simulink model "EHB_speedgoat_R2020a_V1"  (R2020a)
settings: Solver=FixedStepDiscrete  StartTime=0.0  StopTime=inf  FixedStep=0.001  RelTol=1e-3  EnableMultiTasking=on
model workspace (MAT data in the model file):
  A : Simulink.Signal (value not decoded)
  B : Simulink.Signal (value not decoded)
  C : Simulink.Signal (value not decoded)
  D : Simulink.Signal (value not decoded)
  E : Simulink.Signal (value not decoded)
  calin = [-9.96 -7.98 -5.98 -3.99 -1.994 0 1.995 3.992 5.99 7.98 9.97]
  calout = [-10 -8 -6 -4 -2 0 2 4 6 8 10]
symbols that are objects in the model workspace (value not decoded): C, D
undefined symbols (not defined in the file): Com1, none, ts_IO612
libraries: simulink x1436, xpcethercatlib x1223, yisutbxlib_utilities x256, xpcutilitieslib x156, hdlsllib x145, canmsglib x46, speedgoatlib_IO602_4 x11, speedgoatlib_IO611 x7, slrttcplib x4, CanManageLib x3, slrtlib x3, xpcseriallib x2
(part 30 of 30)

== system EHB_speedgoat_R2020a_V1/保留/YS4008/YS4008_M_6/YS4008_M/FIU_CH6/Protect ==
  KL30_In : Inport
  KL31_In : Inport  Port=2
  COM_In : Inport  Port=3
  Open_In : Inport  Port=4
  Compare To Constant{,2,12,14} (4 alike) : simulink/Logic and Bit Operations/Compare To Constant  relop===  const=1  OutDataTypeStr=boolean
  Compare To Constant{1,3..11,13,15} (12 alike) : simulink/Logic and Bit Operations/Compare To Constant  relop===  const=0  OutDataTypeStr=boolean
  Logical Operator{,1..3} (4 alike) : Logic  Inputs=4  AllPortsSameDT=off  OutDataTypeStr=boolean
  KL30_Out : Outport
  KL31_Out : Outport  Port=2
  COM_Out : Outport  Port=3
  Open_Out : Outport  Port=4
  wires:
  [Open_In] -> Compare To Constant14/1
  [COM_In] -> Compare To Constant13/1
  [KL31_In] -> Compare To Constant10/1
  [KL30_In] -> Compare To Constant8/1
  [Open_In] -> Compare To Constant15/1
  [COM_In] -> Compare To Constant12/1
  [KL31_In] -> Compare To Constant11/1
  [KL30_In] -> Compare To Constant7/1
  [COM_In] -> Compare To Constant5/1
  [KL31_In] -> Compare To Constant2/1
  [KL30_In] -> Compare To Constant1/1
  [Open_In] -> Compare To Constant6/1
  [COM_In] -> Compare To Constant4/1
  [KL31_In] -> Compare To Constant3/1
  [KL30_In] -> Compare To Constant/1
  [Open_In] -> Compare To Constant9/1
  Logical Operator/1 -> [KL30_Out]
  Logical Operator3/1 -> [Open_Out]
  Logical Operator2/1 -> [COM_Out]
  Logical Operator1/1 -> [KL31_Out]
  [Open_Out] -> Open_Out/1
  Compare To Constant7/1 -> Logical Operator2/1
  Compare To Constant11/1 -> Logical Operator2/2
  Compare To Constant12/1 -> Logical Operator2/3
  Compare To Constant15/1 -> Logical Operator2/4
  Compare To Constant14/1 -> Logical Operator3/4
  Compare To Constant13/1 -> Logical Operator3/3
  Compare To Constant10/1 -> Logical Operator3/2
  Compare To Constant8/1 -> Logical Operator3/1
  Compare To Constant1/1 -> Logical Operator1/1
  Compare To Constant2/1 -> Logical Operator1/2
  Compare To Constant5/1 -> Logical Operator1/3
  Compare To Constant6/1 -> Logical Operator1/4
  Compare To Constant9/1 -> Logical Operator/4
  Open_In/1 -> [Open_In]
  [KL31_Out] -> KL31_Out/1
  [KL30_Out] -> KL30_Out/1
  [COM_Out] -> COM_Out/1
  Compare To Constant4/1 -> Logical Operator/3
  Compare To Constant3/1 -> Logical Operator/2
  KL31_In/1 -> [KL31_In]
  KL30_In/1 -> [KL30_In]
  COM_In/1 -> [COM_In]
  Compare To Constant/1 -> Logical Operator/1

== system EHB_speedgoat_R2020a_V1/保留/YS4008/YS4008_M_6/YS4008_M/FIU_CH7/Protect ==
  KL30_In : Inport
  KL31_In : Inport  Port=2
  COM_In : Inport  Port=3
  Open_In : Inport  Port=4
  Compare To Constant{,2,12,14} (4 alike) : simulink/Logic and Bit Operations/Compare To Constant  relop===  const=1  OutDataTypeStr=boolean
  Compare To Constant{1,3..11,13,15} (12 alike) : simulink/Logic and Bit Operations/Compare To Constant  relop===  const=0  OutDataTypeStr=boolean
  Logical Operator{,1..3} (4 alike) : Logic  Inputs=4  AllPortsSameDT=off  OutDataTypeStr=boolean
  KL30_Out : Outport
  KL31_Out : Outport  Port=2
  COM_Out : Outport  Port=3
  Open_Out : Outport  Port=4
  wires:
  Compare To Constant/1 -> Logical Operator/1
  COM_In/1 -> [COM_In]
  KL30_In/1 -> [KL30_In]
  KL31_In/1 -> [KL31_In]
  Compare To Constant3/1 -> Logical Operator/2
  Compare To Constant4/1 -> Logical Operator/3
  [COM_Out] -> COM_Out/1
  [KL30_Out] -> KL30_Out/1
  [KL31_Out] -> KL31_Out/1
  Open_In/1 -> [Open_In]
  Compare To Constant9/1 -> Logical Operator/4
  Compare To Constant6/1 -> Logical Operator1/4
  Compare To Constant5/1 -> Logical Operator1/3
  Compare To Constant2/1 -> Logical Operator1/2
  Compare To Constant1/1 -> Logical Operator1/1
  Compare To Constant8/1 -> Logical Operator3/1
  Compare To Constant10/1 -> Logical Operator3/2
  Compare To Constant13/1 -> Logical Operator3/3
  Compare To Constant14/1 -> Logical Operator3/4
  Compare To Constant15/1 -> Logical Operator2/4
  Compare To Constant12/1 -> Logical Operator2/3
  Compare To Constant11/1 -> Logical Operator2/2
  Compare To Constant7/1 -> Logical Operator2/1
  [Open_Out] -> Open_Out/1
  Logical Operator1/1 -> [KL31_Out]
  Logical Operator2/1 -> [COM_Out]
  Logical Operator3/1 -> [Open_Out]
  Logical Operator/1 -> [KL30_Out]
  [Open_In] -> Compare To Constant9/1
  [KL30_In] -> Compare To Constant/1
  [KL31_In] -> Compare To Constant3/1
  [COM_In] -> Compare To Constant4/1
  [Open_In] -> Compare To Constant6/1
  [KL30_In] -> Compare To Constant1/1
  [KL31_In] -> Compare To Constant2/1
  [COM_In] -> Compare To Constant5/1
  [KL30_In] -> Compare To Constant7/1
  [KL31_In] -> Compare To Constant11/1
  [COM_In] -> Compare To Constant12/1
  [Open_In] -> Compare To Constant15/1
  [KL30_In] -> Compare To Constant8/1
  [KL31_In] -> Compare To Constant10/1
  [COM_In] -> Compare To Constant13/1
  [Open_In] -> Compare To Constant14/1

== system EHB_speedgoat_R2020a_V1/保留/YS4008/YS4008_M_6/YS4008_M/FIU_CH8/Protect ==
  KL30_In : Inport
  KL31_In : Inport  Port=2
  COM_In : Inport  Port=3
  Open_In : Inport  Port=4
  Compare To Constant{,2,12,14} (4 alike) : simulink/Logic and Bit Operations/Compare To Constant  relop===  const=1  OutDataTypeStr=boolean
  Compare To Constant{1,3..11,13,15} (12 alike) : simulink/Logic and Bit Operations/Compare To Constant  relop===  const=0  OutDataTypeStr=boolean
  Logical Operator{,1..3} (4 alike) : Logic  Inputs=4  AllPortsSameDT=off  OutDataTypeStr=boolean
  KL30_Out : Outport
  KL31_Out : Outport  Port=2
  COM_Out : Outport  Port=3
  Open_Out : Outport  Port=4
  wires:
  [Open_In] -> Compare To Constant14/1
  [COM_In] -> Compare To Constant13/1
  [KL31_In] -> Compare To Constant10/1
  [KL30_In] -> Compare To Constant8/1
  [Open_In] -> Compare To Constant15/1
  [COM_In] -> Compare To Constant12/1
  [KL31_In] -> Compare To Constant11/1
  [KL30_In] -> Compare To Constant7/1
  [COM_In] -> Compare To Constant5/1
  [KL31_In] -> Compare To Constant2/1
  [KL30_In] -> Compare To Constant1/1
  [Open_In] -> Compare To Constant6/1
  [COM_In] -> Compare To Constant4/1
  [KL31_In] -> Compare To Constant3/1
  [KL30_In] -> Compare To Constant/1
  [Open_In] -> Compare To Constant9/1
  Logical Operator/1 -> [KL30_Out]
  Logical Operator3/1 -> [Open_Out]
  Logical Operator2/1 -> [COM_Out]
  Logical Operator1/1 -> [KL31_Out]
  [Open_Out] -> Open_Out/1
  Compare To Constant7/1 -> Logical Operator2/1
  Compare To Constant11/1 -> Logical Operator2/2
  Compare To Constant12/1 -> Logical Operator2/3
  Compare To Constant15/1 -> Logical Operator2/4
  Compare To Constant14/1 -> Logical Operator3/4
  Compare To Constant13/1 -> Logical Operator3/3
  Compare To Constant10/1 -> Logical Operator3/2
  Compare To Constant8/1 -> Logical Operator3/1
  Compare To Constant1/1 -> Logical Operator1/1
  Compare To Constant2/1 -> Logical Operator1/2
  Compare To Constant5/1 -> Logical Operator1/3
  Compare To Constant6/1 -> Logical Operator1/4
  Compare To Constant9/1 -> Logical Operator/4
  Open_In/1 -> [Open_In]
  [KL31_Out] -> KL31_Out/1
  [KL30_Out] -> KL30_Out/1
  [COM_Out] -> COM_Out/1
  Compare To Constant4/1 -> Logical Operator/3
  Compare To Constant3/1 -> Logical Operator/2
  KL31_In/1 -> [KL31_In]
  KL30_In/1 -> [KL30_In]
  COM_In/1 -> [COM_In]
  Compare To Constant/1 -> Logical Operator/1

== system EHB_speedgoat_R2020a_V1/保留/YS4008/YS4008_M_6/YS4008_M/FIU_MsgSend/CANDataPack_ToUDP ==
  In1 : Inport
  "Bit Packing " : xpcutilitieslib/Bit Packing   MaskBitPatterns={[7],[6],[4 5],[0:3]}  MaskPackDataType=uint8  MaskPackDataSize=[1]
      settings: SourceProductBaseCode=XP
  Bit Slice : hdlsllib/Logic and Bit Operations/Bit Slice  lidx=3  ridx=0
      settings: SourceProductBaseCode=SL
  Bus Selector : BusSelector  OutputSignals=Extended,Length,Remote,ID,Data
  "Byte Packing " : xpcutilitieslib/Byte Packing   MaskPackedDataType=uint8  MaskUnpackedDataTypes={'uint32'}  MaskAlignment=1
  "Byte Reversal " : xpcutilitieslib/Byte Reversal   numInp=1
      settings: SourceProductBaseCode=XP
  Constant1 : Constant  Value=[0 0]
  Data Type Conversion1 : DataTypeConversion  OutDataTypeStr=boolean
  Data Type Conversion2 : DataTypeConversion  OutDataTypeStr=uint8
  Data Type Conversion9 : DataTypeConversion  OutDataTypeStr=boolean
  Mux : Mux  Inputs=3
  Output : Outport
  wires:
  Bus Selector/5 -> Mux/3  "<Data>"
  "Bit Packing "/1 -> Mux/1  "YS5002_PowerSet"
  Bus Selector/2 -> Data Type Conversion2/1  "<Length>"
  Bus Selector/4 -> "Byte Reversal "/1  "<ID>"
  In1/1 -> Bus Selector/1
  Bus Selector/1 -> Data Type Conversion9/1  "<Extended>"
  Bus Selector/3 -> Data Type Conversion1/1  "<Remote>"
  Data Type Conversion9/1 -> "Bit Packing "/1
  "Byte Reversal "/1 -> "Byte Packing "/1
  Bit Slice/1 -> "Bit Packing "/4
  "Byte Packing "/1 -> Mux/2
  Constant1/1 -> "Bit Packing "/3
  Mux/1 -> Output/1
  Data Type Conversion2/1 -> Bit Slice/1
  Data Type Conversion1/1 -> "Bit Packing "/2
